simulink model "week1_problem5"  (R2020b)
settings: Solver=VariableStepAuto  StartTime=0.0  StopTime=10.0  RelTol=1e-3
model workspace (MAT data in the model file):
  C = 0.1
  R = 10
settings Model: Creator=sai  LastModifiedBy=sai

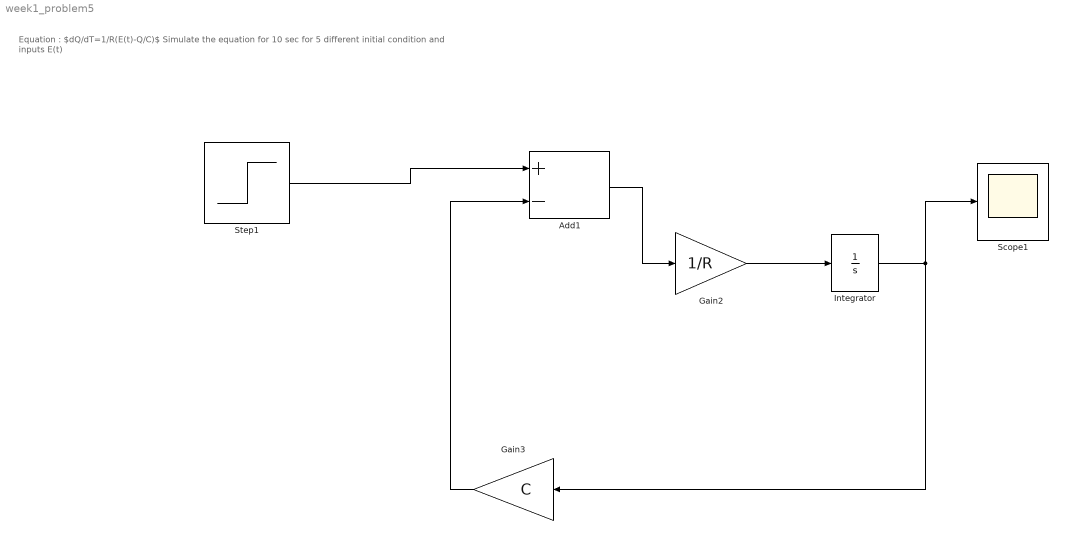
== system week1_problem5 ==
  note: Equation : $dQ/dT=1/R(E(t)-Q/C)$
      | Simulate the equation for 10 sec for 5 different initial condition and inputs E(t)
  Add1 : Sum  Inputs=+-
  Gain2 : Gain  Gain=1/R
  Gain3 : Gain  Gain=C
  Integrator : Integrator
  Scope1 : Scope
  Step1 : Step  Before=2  SampleTime=0
  wires:
  Step1/1 -> Add1/1
  Integrator/1 -> Scope1/1, Gain3/1
  Gain2/1 -> Integrator/1
  Gain3/1 -> Add1/2
  Add1/1 -> Gain2/1
